simulink subsystem "simulation_window_simulink_sub"  (R2022b)
settings: Solver=VariableStepAuto  StartTime=0.0  StopTime=10.0  RelTol=1e-3
settings Model: Creator=User  LastModifiedBy=User

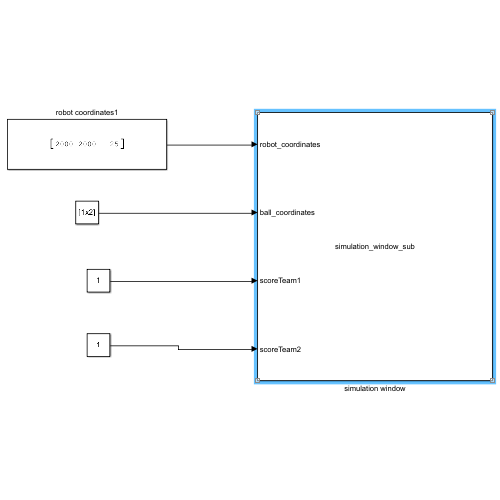
[thumbnail: Simulink's stored preview of the top-level diagram]
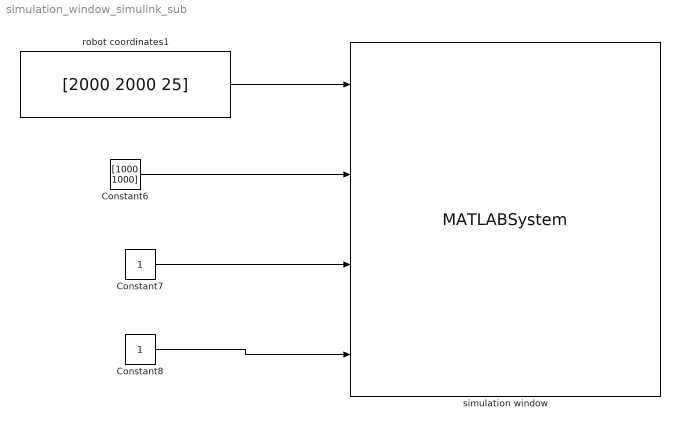
== system simulation_window_simulink_sub ==
  Constant6 : Constant  Value=[1000 1000]
  Constant7 : Constant
  Constant8 : Constant
  robot coordinates1 : Constant  Value=[2000 2000 25]  VectorParams1D=off
  simulation window : MATLABSystem  System=simulation_window_sub  pitch_length=9000  pitch_width=6000  centre_circle_diameter=1500  border_strip_width=1000  goal_area_length=1000  goal_area_width=1000  penalty_area_length=1000  penalty_area_width=3000  goal_width=1000  goal_depth=500  SimulateUsing=Code generation
      mask Type: simulation_window_sub
      mask Display:
      | disp('simulation_window_sub');
      | port_label('input',1,'robot_coordinates');
      | port_label('input',2,'ball_coordinates');
      | port_label('input',3,'scoreTeam1');
      | port_label('input',4,'scoreTeam2');
  wires:
  Constant6/1 -> simulation window/2
  robot coordinates1/1 -> simulation window/1
  Constant7/1 -> simulation window/3
  Constant8/1 -> simulation window/4
